simulink model "ADC"  (R2015a)
settings: Solver=ode45  StartTime=0.0  StopTime=10e-5  RelTol=1e-3
libraries: dsparch4 x1
settings Model: Creator=John  LastModifiedBy=John

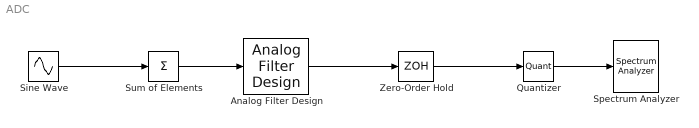
== system ADC ==
  Analog Filter Design : dsparch4/Analog Filter Design  method=Butterworth  filttype=Lowpass  N=8  Wlo=2*pi*50e6  Whi=80  Rp=2  Rs=40
  Quantizer : Quantizer  QuantizationInterval=2^-8
  Sine Wave : Sin  Amplitude=.25  Frequency=2*pi*[20 22]*1e6  SampleTime=0
  Spectrum Analyzer : SpectrumAnalyzer
  Sum of Elements : Sum  Inputs=+
  Zero-Order Hold : ZeroOrderHold  SampleTime=1/100e6
  wires:
  Sine Wave/1 -> Sum of Elements/1
  Sum of Elements/1 -> Analog Filter Design/1
  Analog Filter Design/1 -> Zero-Order Hold/1
  Zero-Order Hold/1 -> Quantizer/1
  Quantizer/1 -> Spectrum Analyzer/1
